simulink model "velo_tc"  (R2015a)
settings: Solver=ode3  StartTime=0.0  StopTime=20.0  RelTol=1e-3
values from neighbouring files (symbols this model uses):
  p_const = 2.5    [k_t_uoffset.m]
  r_const = 1.8    [k_t_uoffset.m]
  s_time = 10    [k_t_uoffset.m]
  u_ini = 2.0    (= 2)    [k_t_uoffset.m]
libraries: arduinolib x2
settings Model: SimulationMode=external  ExtModeTrigDuration=2  Creator=shohei  LastModifiedBy=shohei
settings OptimizationCC: OptimizeModelRefInitCode=on  LifeSpan=1
settings DebuggingCC: UnderspecifiedInitializationDetection=Classic  MergeDetectMultiDrivingBlocksExec=none
settings HardwareCC: ProdBitPerInt=16  ProdBitPerPointer=8  ProdIntDivRoundTo=Zero  ProdEndianess=LittleEndian  ProdWordSize=8  ProdHWDeviceType=Atmel->AVR
settings RTWCC: SystemTargetFile=realtime.tlc  GenerateMakefile=off  TemplateMakefile=realtime.tmf  Description=Run on Target Hardware  RTWVerbose=off
settings ERTTargetCC: CombineOutputUpdateFcns=off  ExtModeTransport=3  ExtModeMexFile=ext_serial_win32_comm_rtt  ExtModeMexArgs=0 1 9600  ERTSrcFileBannerTemplate=realtime_code_template.cgt  ERTHdrFileBannerTemplate=realtime_code_template.cgt  ERTDataSrcFileTemplate=realtime_code_template.cgt  ERTDataHdrFileTemplate=realtime_code_template.cgt  ERTCustomFileTemplate=realtime_file_process.tlc

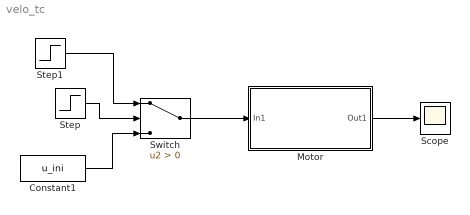
== system velo_tc ==
  Constant1 : Constant  Value=u_ini
  "Motor " : Subsystem
  Scope : Scope
      settings: SaveName=yout
  Step : Step  SampleTime=0
  Step1 : Step  Time=s_time  Before=r_const  After=p_const  SampleTime=0
  Switch : Switch  Criteria=u2 > Threshold
  wires:
  "Motor "/1(Out1) -> Scope/1
  Step/1 -> Switch/2
  Constant1/1 -> Switch/3
  Step1/1 -> Switch/1
  Switch/1 -> "Motor "/1(In1)

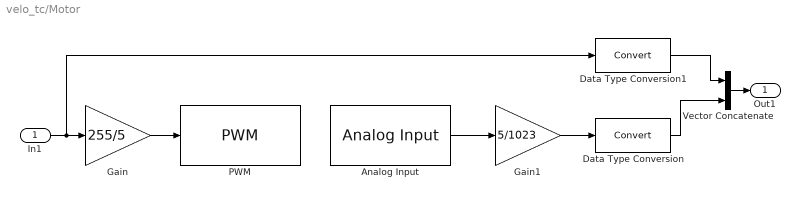
== system velo_tc/Motor  ==
  In1 : Inport
  Analog Input : arduinolib/Analog Input  pinNumber=5  sampleTime=0.01  blockPlatform=arduino
  Data Type Conversion : DataTypeConversion
  Data Type Conversion1 : DataTypeConversion
  Gain : Gain  Gain=255/5
  Gain1 : Gain  Gain=5/1023
  PWM : arduinolib/PWM  pinNumber=9  blockPlatform=arduino
  Vector Concatenate : Concatenate
  Out1 : Outport
  wires:
  Gain/1 -> PWM/1
  Gain1/1 -> Data Type Conversion/1
  Vector Concatenate/1 -> Out1/1
  Analog Input/1 -> Gain1/1
  Data Type Conversion/1 -> Vector Concatenate/2
  In1/1 -> Data Type Conversion1/1, Gain/1
  Data Type Conversion1/1 -> Vector Concatenate/1
